simulink model "PID_d"  (R2016a)
settings: Solver=VariableStepAuto  StartTime=0.0  StopTime=10.0  RelTol=1e-3
undefined symbols (not defined in the file): D_d, I_d, P_d, timestep
settings Model: Creator=mgreiff  LastModifiedBy=mgreiff
settings DataIOCC: LimitDataPoints=on
settings DebuggingCC: AllowSymbolicDim=off
settings ModelReferenceCC: PropagateSignalLabelsOutOfModel=off
settings GRTTargetCC: GeneratePreprocessorConditionals=Use local settings

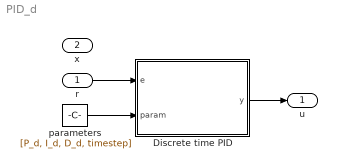
== system PID_d ==
  r : Inport
  x : Inport  Port=2
  Discrete time PID : MATLAB Function  TreatAsAtomicUnit=on
  parameters : Constant  Value=[P_d, I_d, D_d, timestep]
  u : Outport
  wires:
  r/1 -> Discrete time PID/1(e)
  Discrete time PID/1(y) -> u/1
  parameters/1 -> Discrete time PID/2(param)

== matlab function PID_d/Discrete time PID ==
  data: e input; y output; param input
function y = PID_d(e, param)
%#codegen
Kp = param(1); Ki = param(2); Kd = param(3); h = param(4);
persistent I
persistent em1
if isempty(I) || isempty(em1)
    I = 0;
    em1 = 0;
end
P = Kp * e;
I = I + Ki * h * e;
D = Kd * (e - em1)/h;
em1 = e;
y = P + I + D;
